simulink subsystem "SeguimientoMFunction"  (R2023b)
settings: Solver=VariableStepAuto  StartTime=0.0  StopTime=10.0  RelTol=1e-3
settings Model: Creator=pablo  LastModifiedBy=pablo

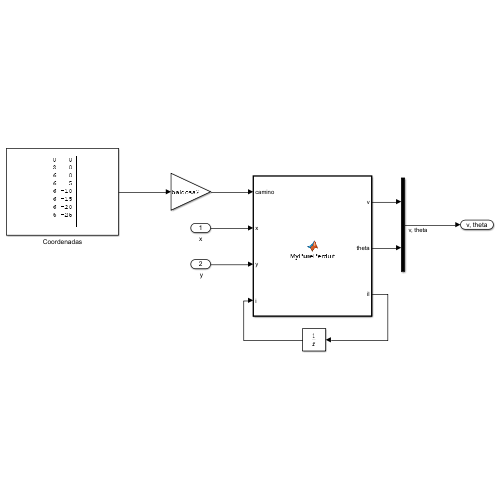
[thumbnail: Simulink's stored preview of the top-level diagram]
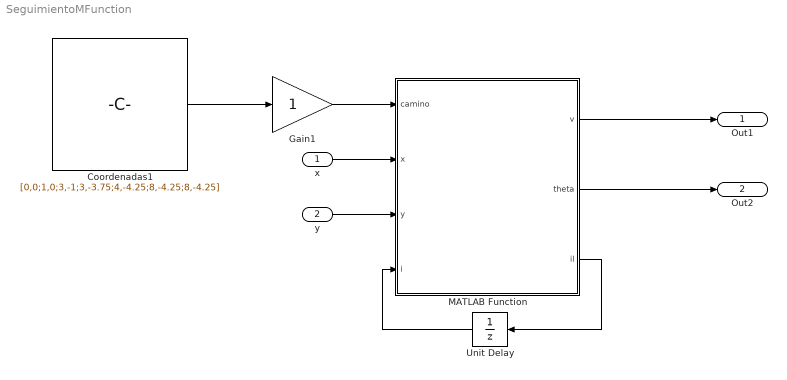
== system SeguimientoMFunction ==
  x : Inport
  " y" : Inport  Port=2
  Coordenadas1 : Constant  Value=[0,0;1,0;3,-1;3,-3.75;4,-4.25;8,-4.25;8,-4.25]
  Gain1 : Gain
  MATLAB Function : MATLAB Function  TreatAsAtomicUnit=on
  Unit Delay : UnitDelay  SampleTime=-1  HasFrameUpgradeWarning=on
  Out1 : Outport
  Out2 : Outport  Port=2
  wires:
  Coordenadas1/1 -> Gain1/1
  MATLAB Function/1(v) -> Out1/1
  x/1 -> MATLAB Function/2(x)
  MATLAB Function/3(il) -> Unit Delay/1
  " y"/1 -> MATLAB Function/3(y)
  Unit Delay/1 -> MATLAB Function/4(i)
  Gain1/1 -> MATLAB Function/1(camino)
  MATLAB Function/2(theta) -> Out2/1

== matlab function SeguimientoMFunction/MATLAB Function ==
  data: camino input; v output; x input; y input; i input; theta output; il output
function [v,theta,il] = MyPurePerduit(camino,x,y,i)
L = 0.05; %Distancia de persecucion
v = 0.205;
i = i+1;
if length(camino)>i %Mientras haya camino
    %Calculamos distancia al objetivo
    distancia = sqrt((camino(i,1)-x)^2 + (camino(i,2)-y)^2);
    while(distancia<L)&&(length(camino)>i) %ya hemos
        i = i + 1; %Actualizar objetivo
        distancia = sqrt((camino(i,1)-x)^2 + (camino(i,2)-y)^2);
        v=0.205;
    end
    %Calculo de la orientacion al punto i-esimo
    theta = atan2((camino(i,2)-y),(camino(i,1)-x));
else %Si ha llegado al objetivo final se para
    theta = 0;
    v = 0;
end

if i<(length(camino))
    il = i -1;
else
    il = i;
end
end
